simulink model "frequence_response_4"  (R2021b)
settings: Solver=VariableStepAuto  StartTime=0.0  StopTime=80  RelTol=1e-3
undefined symbols (not defined in the file or in its folder): A, B, C, D
settings Model: Creator=PaoloA  LastModifiedBy=PaoloA

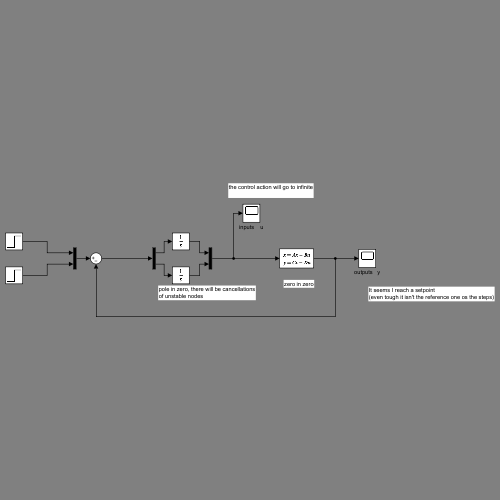
[thumbnail: Simulink's stored preview of the top-level diagram]
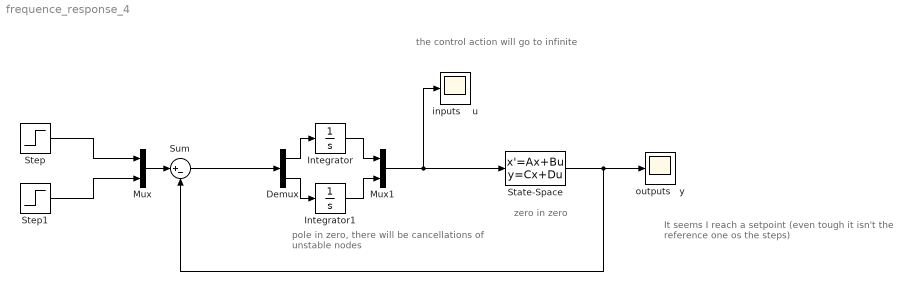
== system frequence_response_4 ==
  note: pole in zero, there will be cancellations
      | of unstable nodes
  note: zero in zero
  note: the control action will go to infinite
  note: It seems I reach a setpoint
      | (even tough it isn't the reference one os the steps)
  Demux : Demux  Outputs=2
  Integrator : Integrator
  Integrator1 : Integrator
  Mux : Mux  Inputs=2
  Mux1 : Mux  Inputs=2
  State-Space : StateSpace  A=A  B=B  C=C  D=D  InitialCondition=0
  Step : Step  Time=2  After=4  SampleTime=0
  Step1 : Step  Time=10  After=6  SampleTime=0
  Sum : Sum  Inputs=|+-
  inputs    u : Scope
  outputs   y : Scope
  wires:
  State-Space/1 -> Sum/2, outputs   y/1
  Step/1 -> Mux/1
  Step1/1 -> Mux/2
  Mux/1 -> Sum/1
  Demux/1 -> Integrator/1
  Integrator/1 -> Mux1/1
  Integrator1/1 -> Mux1/2
  Demux/2 -> Integrator1/1
  Mux1/1 -> inputs    u/1, State-Space/1
  Sum/1 -> Demux/1
